simulink model "Commander"  (R2025b)
settings: Solver=FixedStepDiscrete  StartTime=0.0  StopTime=inf  FixedStep=0.1  RelTol=1e-3
StartFcn:
  | commanderCommandAuditStep('reset');
settings Model: DataDictionary=CommandDict.sldd  Creator=89447  LastModifiedBy=89447
settings OptimizationCC: DefaultParameterBehavior=Inlined  EnhancedBackFolding=on  PassReuseOutputArgsAs=Individual arguments  ZeroExternalMemoryAtStartup=off  ZeroInternalMemoryAtStartup=off  MaxStackSize=64  OptimizeBlockOrder=speed  DifferentSizesBufferReuse=on  OptimizationCustomize=off  EfficientTunableParamExpr=on
settings HardwareCC: ProdBitPerLong=64.0  ProdHWDeviceType=Intel->x86-64 (Linux 64)  TargetBitPerLong=64.0  TargetBitPerPointer=64.0  TargetBitPerSizeT=64.0  TargetBitPerPtrDiffT=64.0  TargetLargestAtomicFloat=Float  TargetIntDivRoundTo=Zero  TargetEndianess=LittleEndian  TargetWordSize=64.0  TargetHWDeviceType=Intel->x86-64 (Linux 64)  ProdEqTarget=off
settings SFSimCC: MATLABDynamicMemAlloc=off
settings RTWCC: SystemTargetFile=ert.tlc  HardwareBoard=Robot Operating System 2 (ROS 2)  TLCOptions="-aInlineSetEventsForThisBaseRateFcn=TLC_FALSE -aSuppressMultiTaskScheduler=TLC_FALSE  -aRateBasedStepFcn=0"  TemplateMakefile=ert_default_tmf  Toolchain=Colcon Tools  TargetLang=C++  Description=Embedded Coder
settings CodeAppCC: ForceParamTrailComments=on  IgnoreCustomStorageClasses=off  OperatorAnnotations=on  SimulinkDataObjDesc=on  SFDataObjDesc=on  InsertBlockDesc=on
settings ERTTargetCC: ExtModeTransport=2.0  ExtModeStaticAlloc=on  ExtModeMexFile=ext_xcp  ExtModeIntrfLevel=Level2 - Open  ERTCustomFileTemplate=example_file_process.tlc  TargetLangStandard=C++11 (ISO)  SupportContinuousTime=on

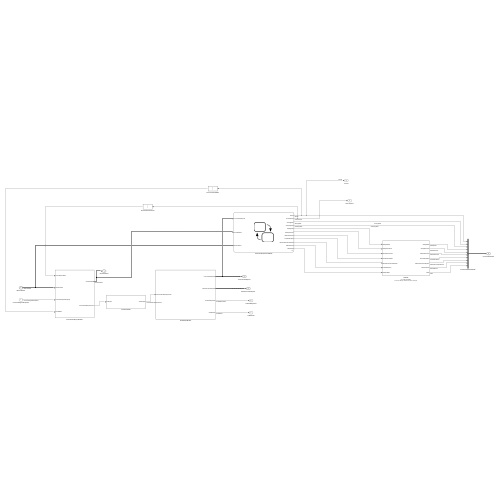
[thumbnail: Simulink's stored preview of the top-level diagram]
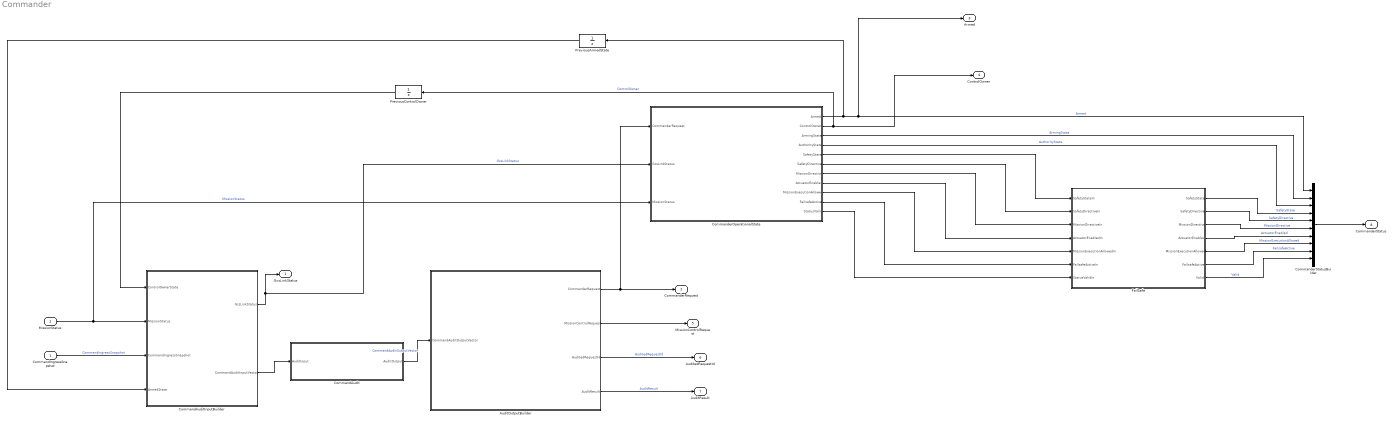
== system Commander ==
  CommandIngressSnapshot : Inport  OutDataTypeStr=double  PortDimensions=17
  MissionStatus : Inport  Port=2  OutDataTypeStr=Bus: MissionStatusBus
  AuditOutputBuilder : Subsystem
  CommandAudit : Subsystem
  CommandAuditInputBuilder : Subsystem
  CommanderOperationalState : Stateflow chart  TreatAsAtomicUnit=on
  CommanderStatusBuilder : BusCreator  Inputs=10  OutDataTypeStr=Bus: CommanderStatusBus
  FailSafe : Subsystem  Description=PLACEHOLDER: preserves the Commander-to-FailSafe architectural boundary while passing through the current CommanderOperationalState safety decisions. Replace this subsystem with the production FailSafe policy/execution adapter without changing CommanderStatusBus.
      settings: AttributesFormatString=|
      | PLACEHOLDER
      | Current safety decisions pass through
  PreviousArmedState : UnitDelay  InitialCondition=false  SampleTime=-1
  PreviousControlOwner : UnitDelay  InitialCondition=uint8(0)  SampleTime=-1
  GcsLinkStatus : Outport  OutDataTypeStr=Bus: GcsLinkStatusBus  BusOutputAsStruct=on
  CommanderRequest : Outport  Port=2  OutDataTypeStr=Bus: CommanderRequestBus  BusOutputAsStruct=on
  Armed : Outport  Port=3  OutDataTypeStr=boolean
  ControlOwner : Outport  Port=4  OutDataTypeStr=uint8
  MissionControlRequest : Outport  Port=5  OutDataTypeStr=Bus: MissionControlRequestBus
  AuditedRequestId : Outport  Port=6
  AuditResult : Outport  Port=7
  CommanderStatus : Outport  Port=8  OutDataTypeStr=Bus: CommanderStatusBus
  wires:
  MissionStatus/1 -> CommanderOperationalState/3(MissionStatus), CommandAuditInputBuilder/2(MissionStatus)  "MissionStatus"
  CommandAuditInputBuilder/1(GcsLinkStatus) -> CommanderOperationalState/2(GcsLinkStatus), GcsLinkStatus/1  "GcsLinkStatus"
  CommandAuditInputBuilder/2(CommandAuditInputVector) -> CommandAudit/1(AuditInput)
  CommandAudit/1(AuditOutput) -> AuditOutputBuilder/1(CommandAuditOutputVector)  "CommandAuditOutputVector"
  AuditOutputBuilder/1(CommanderRequest) -> CommanderRequest/1, CommanderOperationalState/1(CommanderRequest)
  AuditOutputBuilder/2(MissionControlRequest) -> MissionControlRequest/1
  CommandIngressSnapshot/1 -> CommandAuditInputBuilder/3(CommandIngressSnapshot)  "CommandIngressSnapshot"
  AuditOutputBuilder/3(AuditedRequestId) -> AuditedRequestId/1  "AuditedRequestId"
  AuditOutputBuilder/4(AuditResult) -> AuditResult/1  "AuditResult"
  CommanderStatusBuilder/1 -> CommanderStatus/1
  CommanderOperationalState/1(Armed) -> Armed/1, CommanderStatusBuilder/1, PreviousArmedState/1  "Armed"
  CommanderOperationalState/2(ControlOwner) -> PreviousControlOwner/1, ControlOwner/1  "ControlOwner"
  CommanderOperationalState/3(ArmingState) -> CommanderStatusBuilder/2  "ArmingState"
  CommanderOperationalState/4(AuthorityState) -> CommanderStatusBuilder/3  "AuthorityState"
  CommanderOperationalState/5(SafetyState) -> FailSafe/1(SafetyStateIn)
  CommanderOperationalState/6(SafetyDirective) -> FailSafe/2(SafetyDirectiveIn)
  CommanderOperationalState/7(MissionDirective) -> FailSafe/3(MissionDirectiveIn)
  CommanderOperationalState/8(ActuatorEnabled) -> FailSafe/4(ActuatorEnabledIn)
  CommanderOperationalState/9(MissionExecutionAllowed) -> FailSafe/5(MissionExecutionAllowedIn)
  CommanderOperationalState/10(FailsafeActive) -> FailSafe/6(FailsafeActiveIn)
  CommanderOperationalState/11(StatusValid) -> FailSafe/7(StatusValidIn)
  PreviousArmedState/1 -> CommandAuditInputBuilder/4(ArmedState)
  PreviousControlOwner/1 -> CommandAuditInputBuilder/1(ControlOwnerState)
  FailSafe/1(SafetyState) -> CommanderStatusBuilder/4  "SafetyState"
  FailSafe/2(SafetyDirective) -> CommanderStatusBuilder/5  "SafetyDirective"
  FailSafe/3(MissionDirective) -> CommanderStatusBuilder/6  "MissionDirective"
  FailSafe/4(ActuatorEnabled) -> CommanderStatusBuilder/7  "ActuatorEnabled"
  FailSafe/5(MissionExecutionAllowed) -> CommanderStatusBuilder/8  "MissionExecutionAllowed"
  FailSafe/6(FailsafeActive) -> CommanderStatusBuilder/9  "FailsafeActive"
  FailSafe/7(Valid) -> CommanderStatusBuilder/10  "Valid"

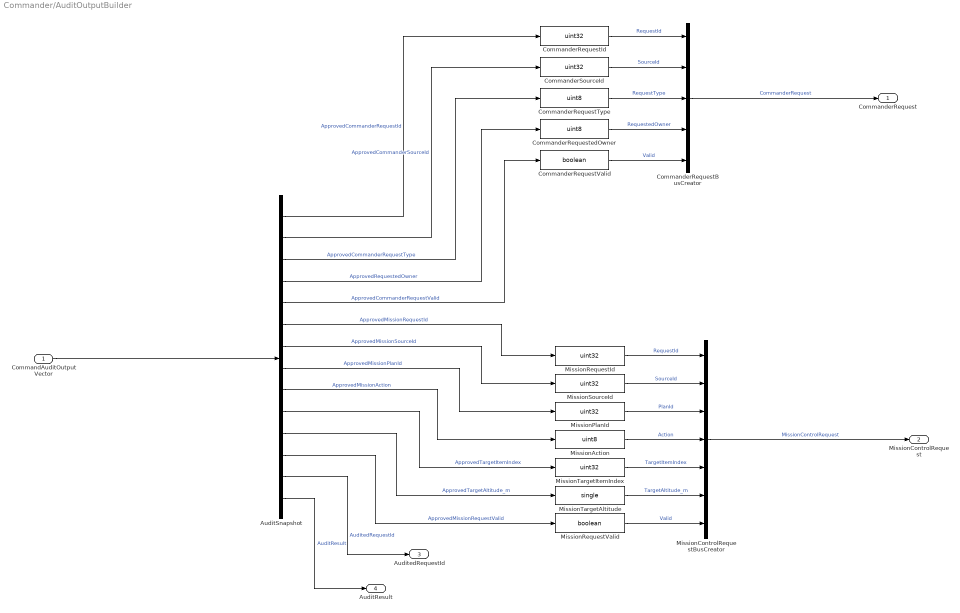
== system Commander/AuditOutputBuilder ==
  CommandAuditOutputVector : Inport
  AuditSnapshot : Demux  Outputs=14
  CommanderRequestBusCreator : BusCreator  Inputs=5  OutDataTypeStr=Bus: CommanderRequestBus  NonVirtualBus=on
  CommanderRequestId : DataTypeConversion  OutDataTypeStr=uint32
  CommanderRequestType : DataTypeConversion  OutDataTypeStr=uint8
  CommanderRequestValid : DataTypeConversion  OutDataTypeStr=boolean
  CommanderRequestedOwner : DataTypeConversion  OutDataTypeStr=uint8
  CommanderSourceId : DataTypeConversion  OutDataTypeStr=uint32
  MissionAction : DataTypeConversion  OutDataTypeStr=uint8
  MissionControlRequestBusCreator : BusCreator  Inputs=7  OutDataTypeStr=Bus: MissionControlRequestBus  NonVirtualBus=on
  MissionPlanId : DataTypeConversion  OutDataTypeStr=uint32
  MissionRequestId : DataTypeConversion  OutDataTypeStr=uint32
  MissionRequestValid : DataTypeConversion  OutDataTypeStr=boolean
  MissionSourceId : DataTypeConversion  OutDataTypeStr=uint32
  MissionTargetAltitude : DataTypeConversion  OutDataTypeStr=single
  MissionTargetItemIndex : DataTypeConversion  OutDataTypeStr=uint32
  CommanderRequest : Outport
  MissionControlRequest : Outport  Port=2
  AuditedRequestId : Outport  Port=3
  AuditResult : Outport  Port=4
  wires:
  AuditSnapshot/13 -> AuditedRequestId/1  "AuditedRequestId"
  MissionRequestValid/1 -> MissionControlRequestBusCreator/7  "Valid"
  CommanderRequestValid/1 -> CommanderRequestBusCreator/5  "Valid"
  AuditSnapshot/11 -> MissionTargetAltitude/1  "ApprovedTargetAltitude_m"
  MissionSourceId/1 -> MissionControlRequestBusCreator/2  "SourceId"
  CommanderRequestType/1 -> CommanderRequestBusCreator/3  "RequestType"
  AuditSnapshot/14 -> AuditResult/1  "AuditResult"
  CommanderRequestId/1 -> CommanderRequestBusCreator/1  "RequestId"
  AuditSnapshot/12 -> MissionRequestValid/1  "ApprovedMissionRequestValid"
  AuditSnapshot/2 -> CommanderSourceId/1  "ApprovedCommanderSourceId"
  AuditSnapshot/5 -> CommanderRequestValid/1  "ApprovedCommanderRequestValid"
  MissionRequestId/1 -> MissionControlRequestBusCreator/1  "RequestId"
  CommandAuditOutputVector/1 -> AuditSnapshot/1
  AuditSnapshot/10 -> MissionTargetItemIndex/1  "ApprovedTargetItemIndex"
  AuditSnapshot/1 -> CommanderRequestId/1  "ApprovedCommanderRequestId"
  AuditSnapshot/3 -> CommanderRequestType/1  "ApprovedCommanderRequestType"
  MissionTargetAltitude/1 -> MissionControlRequestBusCreator/6  "TargetAltitude_m"
  AuditSnapshot/4 -> CommanderRequestedOwner/1  "ApprovedRequestedOwner"
  MissionTargetItemIndex/1 -> MissionControlRequestBusCreator/5  "TargetItemIndex"
  AuditSnapshot/6 -> MissionRequestId/1  "ApprovedMissionRequestId"
  MissionAction/1 -> MissionControlRequestBusCreator/4  "Action"
  AuditSnapshot/7 -> MissionSourceId/1  "ApprovedMissionSourceId"
  AuditSnapshot/8 -> MissionPlanId/1  "ApprovedMissionPlanId"
  CommanderRequestedOwner/1 -> CommanderRequestBusCreator/4  "RequestedOwner"
  CommanderSourceId/1 -> CommanderRequestBusCreator/2  "SourceId"
  AuditSnapshot/9 -> MissionAction/1  "ApprovedMissionAction"
  MissionPlanId/1 -> MissionControlRequestBusCreator/3  "PlanId"
  CommanderRequestBusCreator/1 -> CommanderRequest/1  "CommanderRequest"
  MissionControlRequestBusCreator/1 -> MissionControlRequest/1  "MissionControlRequest"

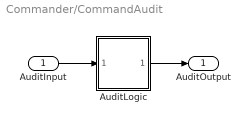
== system Commander/CommandAudit ==
  AuditInput : Inport  PortDimensions=19
  AuditLogic : MATLAB Function  TreatAsAtomicUnit=on
  AuditOutput : Outport  PortDimensions=14
  wires:
  AuditInput/1 -> AuditLogic/1(input)
  AuditLogic/1(output) -> AuditOutput/1

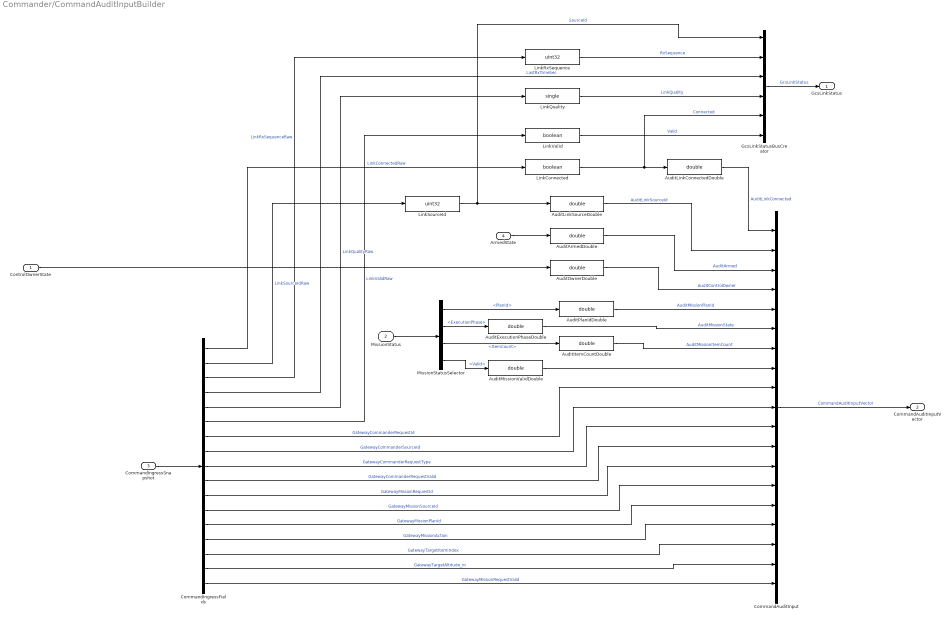
== system Commander/CommandAuditInputBuilder ==
  ControlOwnerState : Inport
  MissionStatus : Inport  Port=2  OutDataTypeStr=Bus: MissionStatusBus
  CommandIngressSnapshot : Inport  Port=3
  ArmedState : Inport  Port=4
  AuditArmedDouble : DataTypeConversion  OutDataTypeStr=double
  AuditExecutionPhaseDouble : DataTypeConversion  OutDataTypeStr=double
  AuditItemCountDouble : DataTypeConversion  OutDataTypeStr=double
  AuditLinkConnectedDouble : DataTypeConversion  OutDataTypeStr=double
  AuditLinkSourceDouble : DataTypeConversion  OutDataTypeStr=double
  AuditMissionValidDouble : DataTypeConversion  OutDataTypeStr=double
  AuditOwnerDouble : DataTypeConversion  OutDataTypeStr=double
  AuditPlanIdDouble : DataTypeConversion  OutDataTypeStr=double
  CommandAuditInput : Mux  Inputs=19
  CommandIngressFields : Demux  Outputs=17
  GcsLinkStatusBusCreator : BusCreator  Inputs=6  OutDataTypeStr=Bus: GcsLinkStatusBus  NonVirtualBus=on
  LinkConnected : DataTypeConversion  OutDataTypeStr=boolean
  LinkQuality : DataTypeConversion  OutDataTypeStr=single
  LinkRxSequence : DataTypeConversion  OutDataTypeStr=uint32
  LinkSourceId : DataTypeConversion  OutDataTypeStr=uint32
  LinkValid : DataTypeConversion  OutDataTypeStr=boolean
  MissionStatusSelector : BusSelector  OutputSignals=PlanId,ExecutionPhase,ItemCount,Valid
  GcsLinkStatus : Outport
  CommandAuditInputVector : Outport  Port=2
  wires:
  AuditItemCountDouble/1 -> CommandAuditInput/7  "AuditMissionItemCount"
  AuditOwnerDouble/1 -> CommandAuditInput/4  "AuditControlOwner"
  CommandIngressFields/7 -> CommandAuditInput/9  "GatewayCommanderRequestId"
  CommandIngressFields/9 -> CommandAuditInput/11  "GatewayCommanderRequestType"
  GcsLinkStatusBusCreator/1 -> GcsLinkStatus/1  "GcsLinkStatus"
  CommandIngressFields/4 -> GcsLinkStatusBusCreator/3  "LastRxTimeSec"
  LinkSourceId/1 -> GcsLinkStatusBusCreator/1, AuditLinkSourceDouble/1  "SourceId"
  MissionStatusSelector/4 -> AuditMissionValidDouble/1  "<Valid>"
  CommandIngressFields/1 -> LinkConnected/1  "LinkConnectedRaw"
  MissionStatusSelector/3 -> AuditItemCountDouble/1  "<ItemCount>"
  CommandAuditInput/1 -> CommandAuditInputVector/1  "CommandAuditInputVector"
  AuditLinkSourceDouble/1 -> CommandAuditInput/2  "AuditLinkSourceId"
  MissionStatusSelector/2 -> AuditExecutionPhaseDouble/1  "<ExecutionPhase>"
  AuditPlanIdDouble/1 -> CommandAuditInput/5  "AuditMissionPlanId"
  CommandIngressFields/2 -> LinkSourceId/1  "LinkSourceIdRaw"
  AuditLinkConnectedDouble/1 -> CommandAuditInput/1  "AuditLinkConnected"
  LinkConnected/1 -> AuditLinkConnectedDouble/1, GcsLinkStatusBusCreator/5  "Connected"
  CommandIngressFields/5 -> LinkQuality/1  "LinkQualityRaw"
  AuditExecutionPhaseDouble/1 -> CommandAuditInput/6  "AuditMissionState"
  MissionStatusSelector/1 -> AuditPlanIdDouble/1  "<PlanId>"
  AuditArmedDouble/1 -> CommandAuditInput/3  "AuditArmed"
  LinkValid/1 -> GcsLinkStatusBusCreator/6  "Valid"
  CommandIngressFields/8 -> CommandAuditInput/10  "GatewayCommanderSourceId"
  CommandIngressFields/6 -> LinkValid/1  "LinkValidRaw"
  AuditMissionValidDouble/1 -> CommandAuditInput/8
  LinkQuality/1 -> GcsLinkStatusBusCreator/4  "LinkQuality"
  CommandIngressFields/3 -> LinkRxSequence/1  "LinkRxSequenceRaw"
  MissionStatus/1 -> MissionStatusSelector/1
  ControlOwnerState/1 -> AuditOwnerDouble/1
  LinkRxSequence/1 -> GcsLinkStatusBusCreator/2  "RxSequence"
  ArmedState/1 -> AuditArmedDouble/1
  CommandIngressSnapshot/1 -> CommandIngressFields/1
  CommandIngressFields/10 -> CommandAuditInput/12  "GatewayCommanderRequestValid"
  CommandIngressFields/11 -> CommandAuditInput/13  "GatewayMissionRequestId"
  CommandIngressFields/12 -> CommandAuditInput/14  "GatewayMissionSourceId"
  CommandIngressFields/13 -> CommandAuditInput/15  "GatewayMissionPlanId"
  CommandIngressFields/14 -> CommandAuditInput/16  "GatewayMissionAction"
  CommandIngressFields/15 -> CommandAuditInput/17  "GatewayTargetItemIndex"
  CommandIngressFields/16 -> CommandAuditInput/18  "GatewayTargetAltitude_m"
  CommandIngressFields/17 -> CommandAuditInput/19  "GatewayMissionRequestValid"

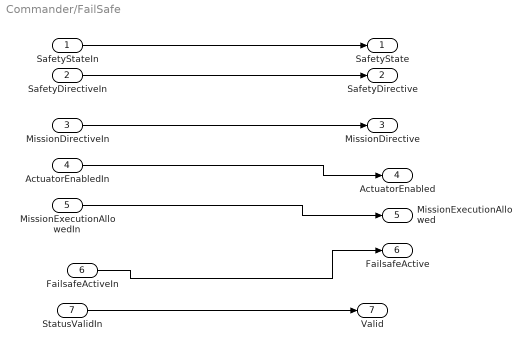
== system Commander/FailSafe ==
  SafetyStateIn : Inport
  SafetyDirectiveIn : Inport  Port=2
  MissionDirectiveIn : Inport  Port=3
  ActuatorEnabledIn : Inport  Port=4
  MissionExecutionAllowedIn : Inport  Port=5
  FailsafeActiveIn : Inport  Port=6
  StatusValidIn : Inport  Port=7
  SafetyState : Outport
  SafetyDirective : Outport  Port=2
  MissionDirective : Outport  Port=3
  ActuatorEnabled : Outport  Port=4
  MissionExecutionAllowed : Outport  Port=5
  FailsafeActive : Outport  Port=6
  Valid : Outport  Port=7
  wires:
  SafetyStateIn/1 -> SafetyState/1
  SafetyDirectiveIn/1 -> SafetyDirective/1
  MissionDirectiveIn/1 -> MissionDirective/1
  ActuatorEnabledIn/1 -> ActuatorEnabled/1
  MissionExecutionAllowedIn/1 -> MissionExecutionAllowed/1
  FailsafeActiveIn/1 -> FailsafeActive/1
  StatusValidIn/1 -> Valid/1

== matlab function Commander/CommandAudit/AuditLogic ==
  data: input input; output output
function output = AuditLogic(input)
%#codegen
output = commanderCommandAuditStep(input);
end

== stateflow chart Commander/CommanderOperationalState ==
  state ArmingRegion [parallel]
    entry:
    Armed = false;
    ArmingState = uint8(0);
    during:
    if CommanderRequest.Valid && CommanderRequest.RequestType == uint8(5)
    ArmingState = uint8(2);
    elseif MissionStatus.Valid && MissionStatus.LandingCompleted
    ArmingState = uint8(0);
    elseif CommanderRequest.Valid && CommanderRequest.RequestType == uint8(4)
    ArmingState = uint8(0);
    elseif ArmingState == uint8(0) && CommanderRequest.Valid && ...
    CommanderRequest.RequestType == uint8(3) && ...
    GcsLinkStatus.Valid && GcsLinkStatus.Connected && ...
    AuthorityState == uint8(1) && SafetyState < uint8(2)
    ArmingState = uint8(1);
    end
    Armed = ArmingState == uint8(1);
    settings: executionOrder=1
  state AuthorityRegion [parallel]
    entry:
    ControlOwner = uint8(0);
    AuthorityState = uint8(0);
    during:
    if GcsLinkStatus.Valid && GcsLinkStatus.Connected
    ControlOwner = uint8(1);
    AuthorityState = uint8(1);
    else
    ControlOwner = uint8(0);
    AuthorityState = uint8(0);
    end
    settings: executionOrder=2
  state SafetyRegion [parallel]
    entry:
    SafetyState = uint8(0);
    during:
    if SafetyState == uint8(3) || CommanderRequest.Valid && ...
    CommanderRequest.RequestType == uint8(5)
    SafetyState = uint8(3);
    elseif MissionStatus.Valid && MissionStatus.MissionFaultCode ~= uint16(0)
    SafetyState = uint8(2);
    elseif Armed && (~GcsLinkStatus.Valid || ~GcsLinkStatus.Connected)
    SafetyState = uint8(2);
    elseif ~GcsLinkStatus.Valid || ~GcsLinkStatus.Connected
    SafetyState = uint8(1);
    else
    SafetyState = uint8(0);
    end
    settings: executionOrder=3
  state DecisionRegion [parallel]
    entry:
    StatusValid = true;
    during:
    StatusValid = true;
    FailsafeActive = SafetyState >= uint8(2);
    ActuatorEnabled = Armed && SafetyState ~= uint8(3);
    MissionExecutionAllowed = Armed && ...
    AuthorityState == uint8(1) && SafetyState == uint8(0) && ...
    GcsLinkStatus.Valid && GcsLinkStatus.Connected;
    if SafetyState == uint8(3)
    SafetyDirective = uint8(4);
    MissionDirective = uint8(2);
    elseif SafetyState == uint8(2) && MissionStatus.Valid && ...
    MissionStatus.MissionFaultCode ~= uint16(0)
    SafetyDirective = uint8(3);
    MissionDirective = uint8(2);
    elseif SafetyState == uint8(2)
    SafetyDirective = uint8(1);
    MissionDirective = uint8(1);
    else
    SafetyDirective = uint8(0);
    MissionDirective = uint8(0);
    end
    settings: executionOrder=4
  data: CommanderRequest input Bus: CommanderRequestBus; GcsLinkStatus input Bus: GcsLinkStatusBus; MissionStatus input Bus: MissionStatusBus; Armed output boolean; ControlOwner output uint8; ArmingState output uint8; AuthorityState output uint8; SafetyState output uint8; SafetyDirective output uint8; MissionDirective output uint8; ActuatorEnabled output boolean; MissionExecutionAllowed output boolean; FailsafeActive output boolean; StatusValid output boolean
